simulink model "NEAT_NN_Par_Controller_3"  (R2018a)
settings: Solver=VariableStepAuto  StartTime=0.0  StopTime=10  RelTol=1e-3  EnableMultiTasking=on
values from neighbouring files (symbols this model uses):
  number_connections = (length(vector_connected_input_nodes)+1)*number_output_nodes    [initial_population.m]    (also in neat_main.m; xor_experiment_vec.m = size(population(index_individual).connectiongenes,2))
  number_nodes = size(population(index_individual).nodegenes,2)    [xor_experiment_vec.m]
undefined symbols (not defined in the file or in its folder): connectiongenes, nodegenes
libraries: aerolibactuator x2, shared3dof x1
settings Model: Creator=arita  LastModifiedBy=arita
settings DataIOCC: LimitDataPoints=on
settings OptimizationCC: LifeSpan=inf
settings DebuggingCC: MaxConsecutiveZCsMsg=none  AllowSymbolicDim=off  SFUnexpectedBacktrackingDiag=warning  SFNoUnconditionalDefaultTransitionDiag=warning  SFExecutionAtInitializationDiag=none
settings ModelReferenceCC: PropagateSignalLabelsOutOfModel=off
settings CodeAppCC: StateflowObjectComments=on
settings GRTTargetCC: TargetLangStandard=C89/C90 (ANSI)
settings ConfigComp: CovMetricSettings=dw  CovHtmlReporting=on  CovSaveCumulativeToWorkspaceVar=on  CovSaveSingleToWorkspaceVar=on  CovExternalEMLEnable=off

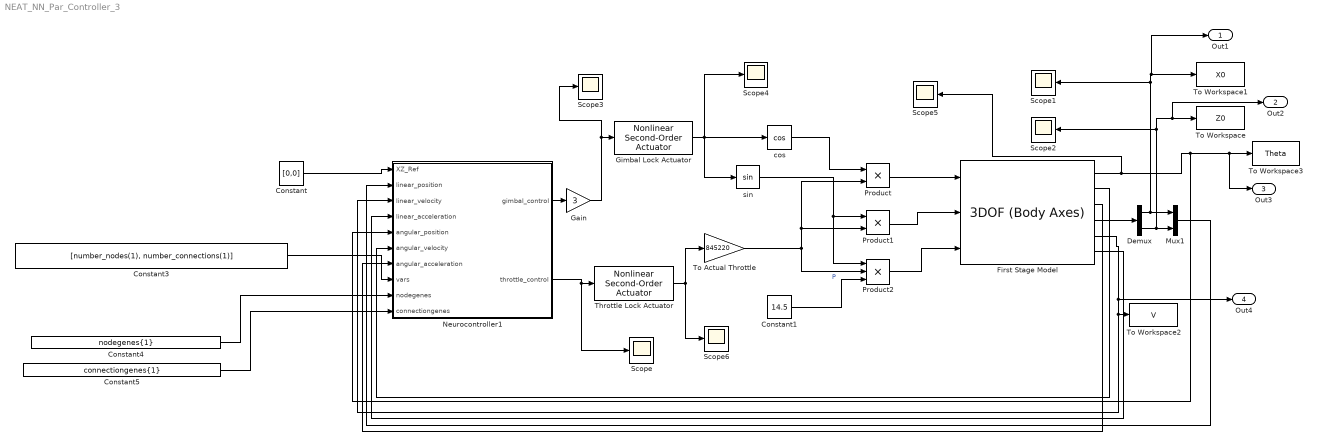
== system NEAT_NN_Par_Controller_3 ==
  Constant : Constant  Value=[0,0]
  Constant1 : Constant  Value=14.5
  Constant3 : Constant  Value=[number_nodes(1), number_connections(1)]
  Constant4 : Constant  Value=nodegenes{1}
  Constant5 : Constant  Value=connectiongenes{1}
  Demux : Demux  Outputs=2
  First Stage Model : shared3dof/3DOF (Body Axes)  units=Metric (MKS)  mtype=Fixed  v_ini=50  theta_ini=90*pi/180  alpha_ini=pi  q_ini=0  pos_ini=[50,-300]  mass=27200  mass_e=0.5  mass_f=3.0  Iyy=3.6244e6  Iyy_e=0.5  Iyy_f=3.0  g_in=Internal  g=9.81  vre_flag=on  abi_flag=off  aMode=aMode
      settings: SourceProductName=Aerospace Blockset  SourceProductBaseCode=AE
  Gain : Gain  Gain=3
  Gimbal Lock Actuator : aerolibactuator/Nonlinear Second-Order Actuator  wn_fin=5  z_fin=1  fin_max=3*pi/180  fin_min=-3*pi/180  fin_maxrate=300  fin_act_0=0  fin_act_vel=0
      settings: SourceProductName=Aerospace Blockset  SourceProductBaseCode=AE
  Mux1 : Mux  Inputs=2
  Neurocontroller1 : MATLAB Function  TreatAsAtomicUnit=on
  Product : Product
  Product1 : Product
  Product2 : Product  Inputs=3
  Scope{,1..6} (7 alike) : Scope
  Throttle Lock Actuator : aerolibactuator/Nonlinear Second-Order Actuator  wn_fin=5  z_fin=1  fin_max=1  fin_min=0  fin_maxrate=300  fin_act_0=0  fin_act_vel=0
      settings: SourceProductName=Aerospace Blockset  SourceProductBaseCode=AE
  To Actual Throttle : Gain  Gain=845220
  To Workspace : ToWorkspace  VariableName=Z0  SaveFormat=Timeseries  SampleTime=0.01
  To Workspace1 : ToWorkspace  VariableName=X0  SaveFormat=Timeseries  SampleTime=0.01
  To Workspace2 : ToWorkspace  VariableName=V  SaveFormat=Timeseries  SampleTime=0.01
  To Workspace3 : ToWorkspace  VariableName=Theta  SaveFormat=Timeseries  SampleTime=0.01
  cos : Trigonometry  Operator=cos
  sin : Trigonometry
  Out1 : Outport
  Out2 : Outport  Port=2
  Out3 : Outport  Port=3
  Out4 : Outport  Port=4
  wires:
  Product/1 -> First Stage Model/1
  sin/1 -> Product1/1, Product2/1
  To Actual Throttle/1 -> Product/2, Product1/2, Product2/2  "P"
  Product1/1 -> First Stage Model/2
  Product2/1 -> First Stage Model/3
  Constant1/1 -> Product2/3
  cos/1 -> Product/1
  Throttle Lock Actuator/1 -> Scope6/1, To Actual Throttle/1
  First Stage Model/4 -> Demux/1
  Demux/1 -> Scope1/1, Out1/1, To Workspace1/1, Mux1/1
  Demux/2 -> Out2/1, To Workspace/1, Scope2/1, Mux1/2
  Neurocontroller1/2(throttle_control) -> Scope/1, Throttle Lock Actuator/1
  Gimbal Lock Actuator/1 -> Scope4/1, sin/1, cos/1
  Constant3/1 -> Neurocontroller1/8(vars)
  Constant4/1 -> Neurocontroller1/9(nodegenes)
  Constant5/1 -> Neurocontroller1/10(connectiongenes)
  Constant/1 -> Neurocontroller1/1(XZ_Ref)
  First Stage Model/1 -> Scope5/1, Neurocontroller1/5(angular_position), Out3/1, To Workspace3/1
  First Stage Model/2 -> Neurocontroller1/6(angular_velocity)
  First Stage Model/3 -> Neurocontroller1/7(angular_acceleration)
  Mux1/1 -> Neurocontroller1/2(linear_position)
  First Stage Model/5 -> Out4/1, Neurocontroller1/3(linear_velocity), To Workspace2/1
  First Stage Model/6 -> Neurocontroller1/4(linear_acceleration)
  Neurocontroller1/1(gimbal_control) -> Gain/1
  Gain/1 -> Scope3/1, Gimbal Lock Actuator/1

== matlab function NEAT_NN_Par_Controller_3/Neurocontroller1 ==
  data: XZ_Ref input; linear_position input; linear_velocity input; linear_acceleration input; angular_position input; angular_velocity input; angular_acceleration input; gimbal_control output; vars input; nodegenes input; connectiongenes input; throttle_control output
function [gimbal_control, throttle_control]  = NN(XZ_Ref, linear_position, linear_velocity, linear_acceleration, angular_position, angular_velocity, angular_acceleration, vars, nodegenes, connectiongenes)
%#codegen
NN_population.nodegenes=nodegenes;
NN_population.connectiongenes=connectiongenes;

number_nodes=vars(1);
number_connections=vars(2);

% change input signals
      NN_population.nodegenes(3,1:2)=XZ_Ref-linear_position; %node input states of the two input nodes are consecutively set to the XOR input pattern  
      NN_population.nodegenes(3,3:4)=linear_velocity;
      NN_population.nodegenes(3,5:6)=linear_acceleration;
      NN_population.nodegenes(3,7)=angular_position;
      NN_population.nodegenes(3,8)=angular_velocity;
      NN_population.nodegenes(3,9)=angular_acceleration;

      
      NN_population.nodegenes(4,1:9)=NN_population.nodegenes(3,1:9);
             
      
         for index_connections=1:number_connections
            %read relevant contents of connection gene (ID of Node where connection starts, ID of Node where it ends, and connection weight)
            ID_connection_from_node=NN_population.connectiongenes(2,index_connections);
            ID_connection_to_node=NN_population.connectiongenes(3,index_connections);
            connection_weight=NN_population.connectiongenes(4,index_connections);
            %map node ID's (as extracted from single connection genes above) to index of corresponding node in node genes matrix
            index_connection_from_node=find((NN_population.nodegenes(1,:)==ID_connection_from_node));
            index_connection_to_node=find((NN_population.nodegenes(1,:)==ID_connection_to_node));
                        
            if NN_population.connectiongenes(5,index_connections)==1 %Check if Connection is enabled
               NN_population.nodegenes(3,index_connection_to_node)=NN_population.nodegenes(3,index_connection_to_node)+NN_population.nodegenes(4,index_connection_from_node)*connection_weight; %take output state of connection_from node, multiply with weight, add to input state of connection_to node
            end
         end
         %pass on node input states to outputs for next timestep 
         NN_population.nodegenes(4,11:number_nodes)=-1+2./(1+exp(-4.9*NN_population.nodegenes(3,11:number_nodes)));          
         %Re-initialize node input states for next timestep
         NN_population.nodegenes(3,11:number_nodes)=0; %set all output and hidden node input states to zero
           gimbal_control = NN_population.nodegenes(4,11);
           throttle_control = NN_population.nodegenes(4,12);
end
